simulink model "az3_forward"  (R2019b)
settings: Solver=VariableStepAuto  StartTime=0.0  StopTime=1.5  RelTol=1e-3
settings Model: Creator=SamRayaneh  LastModifiedBy=SamRayaneh

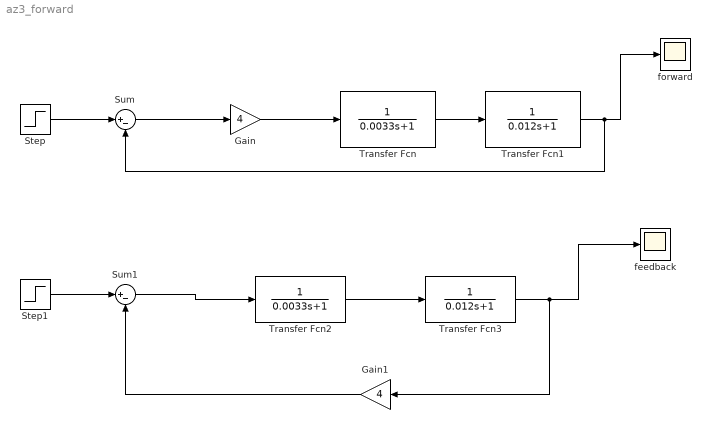
== system az3_forward ==
  Gain : Gain  Gain=4
  Gain1 : Gain  Gain=4
  Step : Step  SampleTime=0
  Step1 : Step  SampleTime=0
  Sum : Sum  Inputs=|+-
  Sum1 : Sum  Inputs=|+-
  Transfer Fcn : TransferFcn  Denominator=[0 0.0033 1]
  Transfer Fcn1 : TransferFcn  Denominator=[0 0.012 1]
  Transfer Fcn2 : TransferFcn  Denominator=[0 0.0033 1]
  Transfer Fcn3 : TransferFcn  Denominator=[0 0.012 1]
  feedback : Scope
  forward : Scope
  wires:
  Step/1 -> Sum/1
  Transfer Fcn/1 -> Transfer Fcn1/1
  Transfer Fcn1/1 -> forward/1, Sum/2
  Gain/1 -> Transfer Fcn/1
  Sum/1 -> Gain/1
  Step1/1 -> Sum1/1
  Sum1/1 -> Transfer Fcn2/1
  Transfer Fcn2/1 -> Transfer Fcn3/1
  Transfer Fcn3/1 -> Gain1/1, feedback/1
  Gain1/1 -> Sum1/2
